simulink library "cav"  (Simulink 8.1)
settings: Solver=ode1  StartTime=0.0  StopTime=Inf  FixedStep=0.001  RelTol=1e-3
PostLoadFcn:
  | , if any(exist('dsrtsu_mdlpostloadfcn', 'file') == [2, 3, 6]), try dsrtsu_mdlpostloadfcn('Execute', bdroot); catch fprintf('Error in PostLoadFcn (dsrtsu_mdlpostloadfcn) for model "%s":\n %s\n', bdroot, lasterr); end, end,
undefined symbols (not defined in the file or in its folder): KJUD_ACCMinActSpeed_kph
libraries: gbp x1
settings Model: DSRTSU_INTERNAL_RTI_VER=450  DSRTSU_INTERNAL_RTI_TYPE=rti1401  RTICANMMDATA=struct('GeneralSetupData',struct('modelroot','D:\ELN150201_TAIWAN\trunk\AdasDragon\software\sw_development\arch\app\jud','generalsettings',struct('filesettings',struct('destfolder',struct('Name','RTICANMM_FILES','Check',1),'buildfolder',struct('Name','.','Check',1),'AbsDestfolder',struct('Name','D:\ELN150201_TAIWAN\trunk\AdasDragon\software\sw_development\arch\app\jud\RTICANMM_FILES'),'AbsBuildfolder',struct('Name','D:\ELN150201_TAIWAN\trunk\AdasDragon\software\sw_development\arch\app\jud'))),'options',struct('addpaths',1,'rmpaths',1,'addtrcexclusion',logical(1),'cannavigator',struct('checkmonitoring',0),'show_usrtrc',0,'use_usrtrc',0),'advanced',struct('options',[1 1 1 1 1 1 1 1 1 1 1 1 1 1 1 1 1 1 1 1 1 1 1 1 1 1 1 1 1 1 1 1 1 1 1 1 1 1 1 1 1 1 1 1 1 1 1 1 1 1 1 1 1 1 1 1 1 1 1 1 1 1 1 1 1 1 1 1 1 1 1 1 1 1 1 1 1 1 1 1 1 1 1 1 1 1 1 1 1 1 1 1 1 1 1 1 1 1 1 1]),'MPSetup',{{}},'modelname','cav','block','cav'))  DSRTSU_INTERNAL_RTIFPGA=40  Creator=AT015411  LastModifiedBy=AT015555

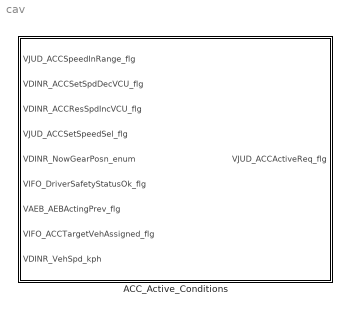
== system cav ==
  ACC_Active_Conditions : Subsystem

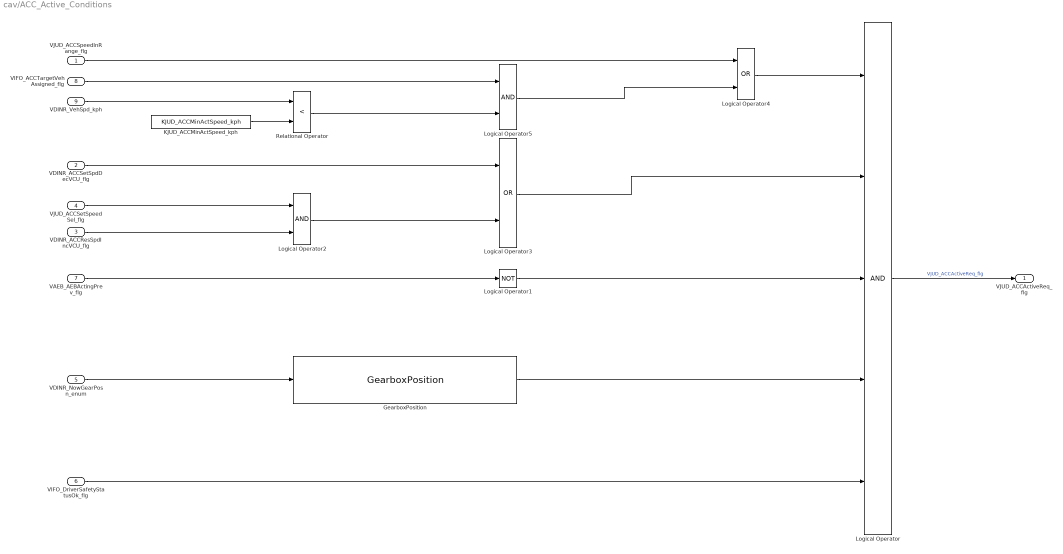
== system cav/ACC_Active_Conditions ==
  VJUD_ACCSpeedInRange_flg : Inport
  VDINR_ACCSetSpdDecVCU_flg : Inport  Port=2
  VDINR_ACCResSpdIncVCU_flg : Inport  Port=3
  VJUD_ACCSetSpeedSel_flg : Inport  Port=4
  VDINR_NowGearPosn_enum : Inport  Port=5
  VIFO_DriverSafetyStatusOk_flg : Inport  Port=6
  VAEB_AEBActingPrev_flg : Inport  Port=7
  VIFO_ACCTargetVehAssigned_flg : Inport  Port=8
  VDINR_VehSpd_kph : Inport  Port=9
  GearboxPosition : gbp/GearboxPosition
  KJUD_ACCMinActSpeed_kph : Constant  Value=KJUD_ACCMinActSpeed_kph
  Logical Operator : Logic  Inputs=5  AllPortsSameDT=off  OutDataTypeStr=boolean
  Logical Operator1 : Logic  Operator=NOT  Inputs=3  AllPortsSameDT=off  OutDataTypeStr=boolean
  Logical Operator2 : Logic  AllPortsSameDT=off  OutDataTypeStr=boolean
  Logical Operator3 : Logic  Operator=OR  AllPortsSameDT=off  OutDataTypeStr=boolean
  Logical Operator4 : Logic  Operator=OR  AllPortsSameDT=off  OutDataTypeStr=boolean
  Logical Operator5 : Logic  AllPortsSameDT=off  OutDataTypeStr=boolean
  Relational Operator : RelationalOperator  Operator=<  OutDataTypeStr=boolean
  VJUD_ACCActiveReq_flg : Outport
  wires:
  Logical Operator/1 -> VJUD_ACCActiveReq_flg/1  "VJUD_ACCActiveReq_flg"
  VAEB_AEBActingPrev_flg/1 -> Logical Operator1/1
  Logical Operator2/1 -> Logical Operator3/2
  VDINR_ACCSetSpdDecVCU_flg/1 -> Logical Operator3/1
  VJUD_ACCSetSpeedSel_flg/1 -> Logical Operator2/1
  VJUD_ACCSpeedInRange_flg/1 -> Logical Operator4/1
  Logical Operator1/1 -> Logical Operator/3
  Logical Operator3/1 -> Logical Operator/2
  VDINR_NowGearPosn_enum/1 -> GearboxPosition/1
  GearboxPosition/1 -> Logical Operator/4
  VIFO_DriverSafetyStatusOk_flg/1 -> Logical Operator/5
  VIFO_ACCTargetVehAssigned_flg/1 -> Logical Operator5/1
  Logical Operator4/1 -> Logical Operator/1
  Logical Operator5/1 -> Logical Operator4/2
  Relational Operator/1 -> Logical Operator5/2
  VDINR_VehSpd_kph/1 -> Relational Operator/1
  KJUD_ACCMinActSpeed_kph/1 -> Relational Operator/2
  VDINR_ACCResSpdIncVCU_flg/1 -> Logical Operator2/2
